simulink model "lab_5_sim"  (R2013a)
settings: Solver=ode45  StartTime=0.0  StopTime=20  RelTol=1e-3  AbsTol=1e-6
undefined symbols (not defined in the file): a, b, c, d, du, t0, u0, x0, x10
settings Model: Creator=LAB320-1552  LastModifiedBy=LAB320-1552
settings DebuggingCC: SolverPrmCheckMsg=none

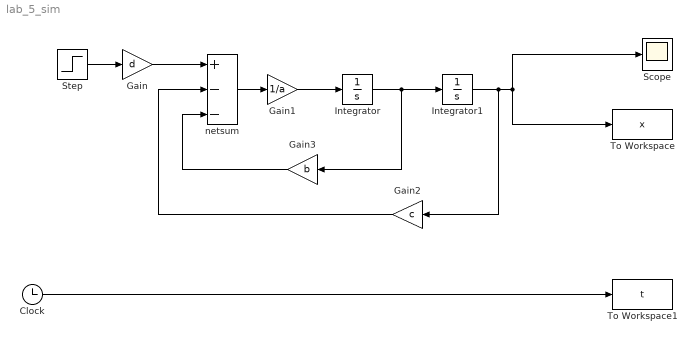
== system lab_5_sim ==
  Clock : Clock
  Gain : Gain  Gain=d
  Gain1 : Gain  Gain=1/a
  Gain2 : Gain  Gain=c
  Gain3 : Gain  Gain=b
  Integrator : Integrator  InitialCondition=x10
  Integrator1 : Integrator  InitialCondition=x0
  Scope : Scope
  Step : Step  Time=t0  Before=u0  After=u0+du  SampleTime=1
  To Workspace : ToWorkspace  VariableName=x  SampleTime=-1
  To Workspace1 : ToWorkspace  VariableName=t  SampleTime=-1
  netsum : Sum  Inputs=+--  SaturateOnIntegerOverflow=on  InputSameDT=on  OutDataTypeStr=Inherit: Same as first input
  wires:
  Step/1 -> Gain/1
  Gain/1 -> netsum/1
  netsum/1 -> Gain1/1
  Integrator/1 -> Gain3/1, Integrator1/1
  Gain3/1 -> netsum/3
  Integrator1/1 -> Gain2/1, Scope/1, To Workspace/1
  Gain2/1 -> netsum/2
  Clock/1 -> To Workspace1/1
  Gain1/1 -> Integrator/1
